simulink subsystem "kalmanFilter"  (R2026a)
settings: Solver=VariableStepAuto
settings Model: Creator=maxhu  LastModifiedBy=maxhu

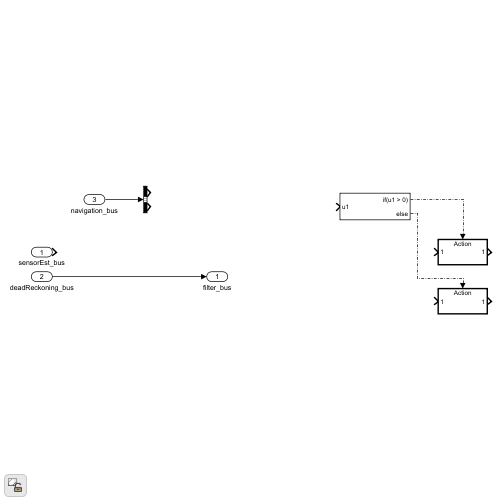
[thumbnail: Simulink's stored preview of the top-level diagram]
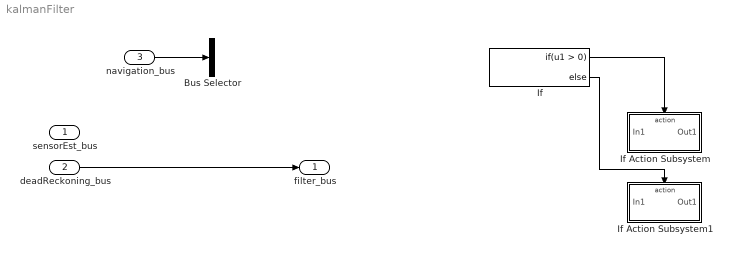
== system kalmanFilter ==
  sensorEst_bus : Inport
  deadReckoning_bus : Inport  Port=2
  navigation_bus : Inport  Port=3
  Bus Selector : BusSelector  OutputSignals=signal1,signal2
  If : If
  If Action Subsystem : Subsystem  TreatAsAtomicUnit=on
  If Action Subsystem1 : Subsystem  TreatAsAtomicUnit=on
  filter_bus : Outport
  wires:
  deadReckoning_bus/1 -> filter_bus/1
  If/1 -> If Action Subsystem/Action
  If/2 -> If Action Subsystem1/Action
  navigation_bus/1 -> Bus Selector/1

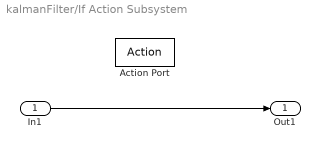
== system kalmanFilter/If Action Subsystem ==
  In1 : Inport
  Action Port : ActionPort
  Out1 : Outport
  wires:
  In1/1 -> Out1/1

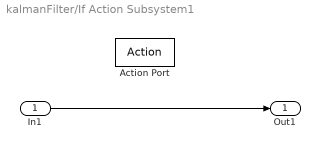
== system kalmanFilter/If Action Subsystem1 ==
  In1 : Inport
  Action Port : ActionPort
  Out1 : Outport
  wires:
  In1/1 -> Out1/1
